simulink model "test"  (R2020a)
settings: Solver=VariableStepAuto  StartTime=0.0  StopTime=inf  RelTol=1e-3
libraries: vrlib x2
settings Model: Creator=sirius  LastModifiedBy=sirius

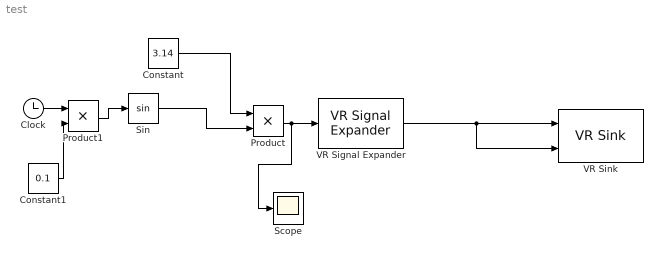
== system test ==
  Clock : Clock
  Constant : Constant  Value=3.14
  Constant1 : Constant  Value=0.1
  Product : Product
  Product1 : Product
  Scope : Scope
  Sin : Trigonometry
  VR Signal Expander : vrlib/VR Signal Expander  outwidth=4  outidx=[4]
  VR Sink : vrlib/VR Sink  InstantiateOnLoad=on  SampleTime=0.1  ViewEnable=on  RemoteChange=off  RemoteView=off  FieldsWritten=Axis_1.rotation.4.1.1.double#Axis_2.rotation.4.1.1.double  WorldFileName=Box.wrl  AutoView=off  VideoDimensions=[]  AllowVariableSize=off
  wires:
  Product/1 -> Scope/1, VR Signal Expander/1
  Sin/1 -> Product/2
  Constant/1 -> Product/1
  Clock/1 -> Product1/1
  Product1/1 -> Sin/1
  Constant1/1 -> Product1/2
  VR Signal Expander/1 -> VR Sink/2, VR Sink/1
